simulink subsystem "OneActuatorAWDSSC"  (R2023a)
settings: Solver=VariableStepAuto  StartTime=0.0  StopTime=10.0  RelTol=1e-3
libraries: fl_lib x2, nesl_utility_internal x1
settings Model: Creator=The MathWorks, Inc.  LastModifiedBy=The MathWorks, Inc.
settings OptimizationCC: ReuseModelBlockBuffer=off

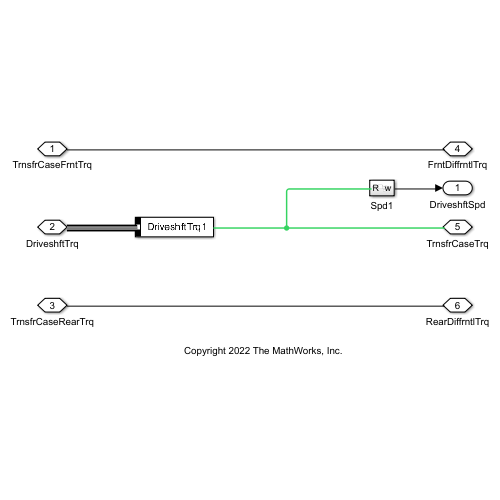
[thumbnail: Simulink's stored preview of the top-level diagram]
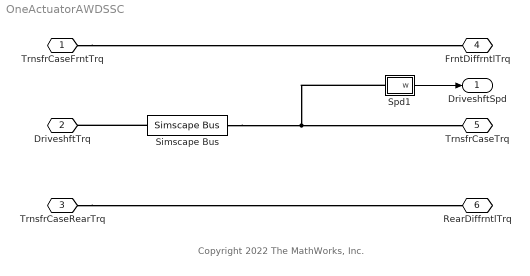
== system OneActuatorAWDSSC ==
  note: Copyright 2022 The MathWorks, Inc.
  Simscape Bus : SimscapeBus  HierarchyStrings=DriveshftTrq1
  Spd1 : Subsystem
  TrnsfrCaseFrntTrq : PMIOPort  Side=Right
  DriveshftTrq : PMIOPort  Port=2  Side=Left
  TrnsfrCaseRearTrq : PMIOPort  Port=3  Side=Right
  FrntDiffrntlTrq : PMIOPort  Port=4  Side=Right
  TrnsfrCaseTrq : PMIOPort  Port=5  Side=Right
  RearDiffrntlTrq : PMIOPort  Port=6  Side=Right
  DriveshftSpd : Outport  VectorParamsAs1DForOutWhenUnconnected=off
  wires:
  Spd1/1(w) -> DriveshftSpd/1
  connections:
  Simscape Bus/LConn1 -- TrnsfrCaseTrq/RConn1 -- Spd1/LConn1
  TrnsfrCaseFrntTrq/RConn1 -- FrntDiffrntlTrq/RConn1
  TrnsfrCaseRearTrq/RConn1 -- RearDiffrntlTrq/RConn1
  Simscape Bus/RConn1 -- DriveshftTrq/RConn1

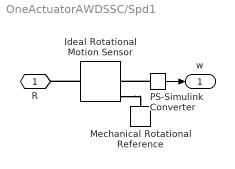
== system OneActuatorAWDSSC/Spd1 ==
  Ideal Rotational Motion Sensor : fl_lib/Mechanical/Mechanical Sensors/Ideal Rotational Motion Sensor  reference=foundation.enum.MeasurementReference.difference  acceleration_port=false  velocity_port=true  position_port=true  wrap_angle=simscape.enum.onoff.off  offset=0 rad
      settings: SourceProductName=Foundation Library
  Mechanical Rotational Reference : fl_lib/Mechanical/Rotational Elements/Mechanical Rotational Reference
      settings: SourceProductName=Foundation Library
  PS-Simulink Converter : nesl_utility_internal/PS-Simulink Converter  PhysicalDomain=network_engine_domain  SubClassName=ps_output  LeftPortType=input  RightPortType=output  PseudoPeriodic=off  Frequencies=[]  VectorFormat=inherit  Unit=inherit  AffineConversion=off
  R : PMIOPort  Side=Left
  w : Outport
  wires:
  PS-Simulink Converter/1 -> w/1
  connections:
  PS-Simulink Converter/LConn1 -- Ideal Rotational Motion Sensor/RConn2
  Ideal Rotational Motion Sensor/LConn1 -- R/RConn1
  Ideal Rotational Motion Sensor/RConn1 -- Mechanical Rotational Reference/LConn1
